simulink model "Resistive_thermal_model"  (R2017a)
settings: Solver=ode45  StartTime=0.0  StopTime=5.0  RelTol=1e-3  EnableMultiTasking=on
values from neighbouring files (symbols this model uses):
  Rth_c1 = 0.00001    (= 1e-05)    [Power_loss_calculation.m]
  Rth_c2 = 0.00001    (= 1e-05)    [Power_loss_calculation.m]
  Rth_c3 = 0.00001    (= 1e-05)    [Power_loss_calculation.m]
  Rth_heatsink = 0.01    [Power_loss_calculation.m]    (also in Thermal_plot.m = [0.005)
  Rth_jc_FWD1L = 0.12    [Power_loss_calculation.m]
  Rth_jc_FWD1U = 0.12    [Power_loss_calculation.m]
  Rth_jc_FWD2L = 0.12    [Power_loss_calculation.m]
  Rth_jc_FWD2U = 0.12    [Power_loss_calculation.m]
  Rth_jc_FWD3L = 0.12    [Power_loss_calculation.m]
  Rth_jc_FWD3U = 0.12    [Power_loss_calculation.m]
  Rth_jc_IGBT1L = 0.066    [Power_loss_calculation.m]
  Rth_jc_IGBT1U = 0.066    [Power_loss_calculation.m]
  Rth_jc_IGBT2L = 0.066    [Power_loss_calculation.m]
  Rth_jc_IGBT2U = 0.066    [Power_loss_calculation.m]
  Rth_jc_IGBT3L = 0.066    [Power_loss_calculation.m]
  Rth_jc_IGBT3U = 0.066    [Power_loss_calculation.m]
  Rth_paste = 0.015    [Power_loss_calculation.m]
libraries: fl_lib x46, nesl_utility x15
settings Model: Creator=Caner  LastModifiedBy=Caner
settings DataIOCC: LimitDataPoints=on  SaveFormat=Array
settings OptimizationCC: LifeSpan=inf
settings DebuggingCC: UnconnectedInputMsg=none  UnconnectedOutputMsg=none  UnconnectedLineMsg=none  SFUnexpectedBacktrackingDiag=warning  SFNoUnconditionalDefaultTransitionDiag=warning  SFExecutionAtInitializationDiag=none
settings HardwareCC: ProdBitPerPointer=32  ProdBitPerSizeT=32  ProdBitPerPtrDiffT=32  ProdLargestAtomicFloat=None  ProdIntDivRoundTo=Undefined  ProdEndianess=Unspecified  ProdWordSize=32  ProdHWDeviceType=32-bit Generic
settings ModelReferenceCC: PropagateSignalLabelsOutOfModel=off
settings GRTTargetCC: TargetLangStandard=C89/C90 (ANSI)  GeneratePreprocessorConditionals=Disable all
settings ConfigComp: CovMetricSettings=dw  CovHtmlReporting=on  CovSaveCumulativeToWorkspaceVar=on  CovSaveSingleToWorkspaceVar=on  CovExternalEMLEnable=off

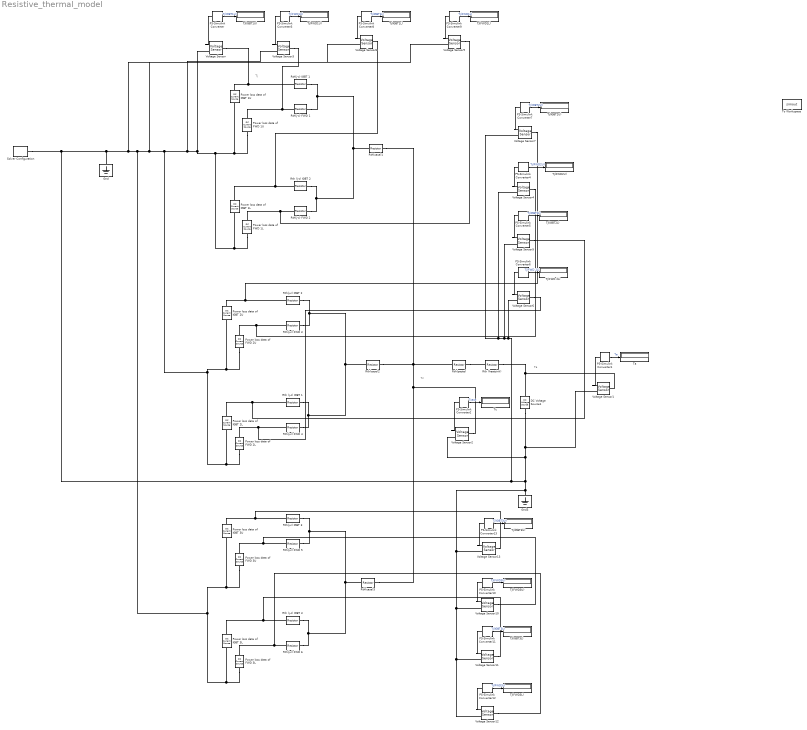
== system Resistive_thermal_model ==
  note: Ta
  note: Tc
  note: Tj
  DC Voltage Source1 : fl_lib/Electrical/Electrical Sources/DC Voltage Source  v0=40 V
  Gnd : fl_lib/Electrical/Electrical Elements/Electrical Reference
  Gnd3 : fl_lib/Electrical/Electrical Elements/Electrical Reference
  PS-Simulink Converter{,1..13} (14 alike) : nesl_utility/PS-Simulink Converter  PhysicalDomain=network_engine_domain  SubClassName=ps_output  LeftPortType=input  RightPortType=output  PseudoPeriodic=off  Frequencies=[]  Unit=1  AffineConversion=off
  Power loss data of FWD 1L : fl_lib/Electrical/Electrical Sources/DC Current Source  i0=PQ A
      settings: SourceProductName=Simscape  SourceProductBaseCode=SS
  Power loss data of FWD 1U : fl_lib/Electrical/Electrical Sources/DC Current Source  i0=PQ A
      settings: SourceProductName=Simscape  SourceProductBaseCode=SS
  Power loss data of FWD 2L : fl_lib/Electrical/Electrical Sources/DC Current Source  i0=PQ A
      settings: SourceProductName=Simscape  SourceProductBaseCode=SS
  Power loss data of FWD 2U : fl_lib/Electrical/Electrical Sources/DC Current Source  i0=PQ A
      settings: SourceProductName=Simscape  SourceProductBaseCode=SS
  Power loss data of FWD 3L : fl_lib/Electrical/Electrical Sources/DC Current Source  i0=PQ A
      settings: SourceProductName=Simscape  SourceProductBaseCode=SS
  Power loss data of FWD 3U : fl_lib/Electrical/Electrical Sources/DC Current Source  i0=PQ A
      settings: SourceProductName=Simscape  SourceProductBaseCode=SS
  Power loss data of IGBT 1L : fl_lib/Electrical/Electrical Sources/DC Current Source  i0=PD A
      settings: SourceProductName=Simscape  SourceProductBaseCode=SS
  Power loss data of IGBT 1U : fl_lib/Electrical/Electrical Sources/DC Current Source  i0=PD A
      settings: SourceProductName=Simscape  SourceProductBaseCode=SS
  Power loss data of IGBT 2L : fl_lib/Electrical/Electrical Sources/DC Current Source  i0=PD A
      settings: SourceProductName=Simscape  SourceProductBaseCode=SS
  Power loss data of IGBT 2U : fl_lib/Electrical/Electrical Sources/DC Current Source  i0=PD A
      settings: SourceProductName=Simscape  SourceProductBaseCode=SS
  Power loss data of IGBT 3L : fl_lib/Electrical/Electrical Sources/DC Current Source  i0=PD A
      settings: SourceProductName=Simscape  SourceProductBaseCode=SS
  Power loss data of IGBT 3U : fl_lib/Electrical/Electrical Sources/DC Current Source  i0=PD A
      settings: SourceProductName=Simscape  SourceProductBaseCode=SS
  Rth (heatsink) : fl_lib/Electrical/Electrical Elements/Resistor  R=Rth_heatsink Ohm  i_specify=off  i_priority=High  i=0 A  i_nominal_specify=off  i_nominal_unit=A  i_nominal_value=1  v_specify=off  v_priority=High  v=0 V  v_nominal_specify=off  v_nominal_unit=V  v_nominal_value=1
  Rth (j-c) IGBT 1 : fl_lib/Electrical/Electrical Elements/Resistor  R=Rth_jc_IGBT2L Ohm  i_specify=off  i_priority=High  i=0 A  i_nominal_specify=off  i_nominal_unit=A  i_nominal_value=1  v_specify=off  v_priority=High  v=0 V  v_nominal_specify=off  v_nominal_unit=V  v_nominal_value=1
  Rth (j-c) IGBT 2 : fl_lib/Electrical/Electrical Elements/Resistor  R=Rth_jc_IGBT1L Ohm  i_specify=off  i_priority=High  i=0 A  i_nominal_specify=off  i_nominal_unit=A  i_nominal_value=1  v_specify=off  v_priority=High  v=0 V  v_nominal_specify=off  v_nominal_unit=V  v_nominal_value=1
  Rth (j-c) IGBT 3 : fl_lib/Electrical/Electrical Elements/Resistor  R=Rth_jc_IGBT3L Ohm  i_specify=off  i_priority=High  i=0 A  i_nominal_specify=off  i_nominal_unit=A  i_nominal_value=1  v_specify=off  v_priority=High  v=0 V  v_nominal_specify=off  v_nominal_unit=V  v_nominal_value=1
  Rth(case)1 : fl_lib/Electrical/Electrical Elements/Resistor  R=Rth_c1 Ohm  i_specify=off  i_priority=High  i=0 A  i_nominal_specify=off  i_nominal_unit=A  i_nominal_value=1  v_specify=off  v_priority=High  v=0 V  v_nominal_specify=off  v_nominal_unit=V  v_nominal_value=1
  Rth(case)2 : fl_lib/Electrical/Electrical Elements/Resistor  R=Rth_c2 Ohm  i_specify=off  i_priority=High  i=0 A  i_nominal_specify=off  i_nominal_unit=A  i_nominal_value=1  v_specify=off  v_priority=High  v=0 V  v_nominal_specify=off  v_nominal_unit=V  v_nominal_value=1
  Rth(case)3 : fl_lib/Electrical/Electrical Elements/Resistor  R=Rth_c3 Ohm  i_specify=off  i_priority=High  i=0 A  i_nominal_specify=off  i_nominal_unit=A  i_nominal_value=1  v_specify=off  v_priority=High  v=0 V  v_nominal_specify=off  v_nominal_unit=V  v_nominal_value=1
  Rth(j-c) FWD 1 : fl_lib/Electrical/Electrical Elements/Resistor  R=Rth_jc_FWD1U Ohm  i_specify=off  i_priority=High  i=0 A  i_nominal_specify=off  i_nominal_unit=A  i_nominal_value=1  v_specify=off  v_priority=High  v=0 V  v_nominal_specify=off  v_nominal_unit=V  v_nominal_value=1
  Rth(j-c) FWD 2 : fl_lib/Electrical/Electrical Elements/Resistor  R=Rth_jc_FWD1L Ohm  i_specify=off  i_priority=High  i=0 A  i_nominal_specify=off  i_nominal_unit=A  i_nominal_value=1  v_specify=off  v_priority=High  v=0 V  v_nominal_specify=off  v_nominal_unit=V  v_nominal_value=1
  Rth(j-c) FWD 3 : fl_lib/Electrical/Electrical Elements/Resistor  R=Rth_jc_FWD2U Ohm  i_specify=off  i_priority=High  i=0 A  i_nominal_specify=off  i_nominal_unit=A  i_nominal_value=1  v_specify=off  v_priority=High  v=0 V  v_nominal_specify=off  v_nominal_unit=V  v_nominal_value=1
  Rth(j-c) FWD 4 : fl_lib/Electrical/Electrical Elements/Resistor  R=Rth_jc_FWD2L Ohm  i_specify=off  i_priority=High  i=0 A  i_nominal_specify=off  i_nominal_unit=A  i_nominal_value=1  v_specify=off  v_priority=High  v=0 V  v_nominal_specify=off  v_nominal_unit=V  v_nominal_value=1
  Rth(j-c) FWD 5 : fl_lib/Electrical/Electrical Elements/Resistor  R=Rth_jc_FWD3U Ohm  i_specify=off  i_priority=High  i=0 A  i_nominal_specify=off  i_nominal_unit=A  i_nominal_value=1  v_specify=off  v_priority=High  v=0 V  v_nominal_specify=off  v_nominal_unit=V  v_nominal_value=1
  Rth(j-c) FWD 6 : fl_lib/Electrical/Electrical Elements/Resistor  R=Rth_jc_FWD3L Ohm  i_specify=off  i_priority=High  i=0 A  i_nominal_specify=off  i_nominal_unit=A  i_nominal_value=1  v_specify=off  v_priority=High  v=0 V  v_nominal_specify=off  v_nominal_unit=V  v_nominal_value=1
  Rth(j-c) IGBT 1 : fl_lib/Electrical/Electrical Elements/Resistor  R=Rth_jc_IGBT1U Ohm  i_specify=off  i_priority=High  i=0 A  i_nominal_specify=off  i_nominal_unit=A  i_nominal_value=1  v_specify=off  v_priority=High  v=0 V  v_nominal_specify=off  v_nominal_unit=V  v_nominal_value=1
  Rth(j-c) IGBT 2 : fl_lib/Electrical/Electrical Elements/Resistor  R=Rth_jc_IGBT2U Ohm  i_specify=off  i_priority=High  i=0 A  i_nominal_specify=off  i_nominal_unit=A  i_nominal_value=1  v_specify=off  v_priority=High  v=0 V  v_nominal_specify=off  v_nominal_unit=V  v_nominal_value=1
  Rth(j-c) IGBT 3 : fl_lib/Electrical/Electrical Elements/Resistor  R=Rth_jc_IGBT3U Ohm  i_specify=off  i_priority=High  i=0 A  i_nominal_specify=off  i_nominal_unit=A  i_nominal_value=1  v_specify=off  v_priority=High  v=0 V  v_nominal_specify=off  v_nominal_unit=V  v_nominal_value=1
  Rth(paste) : fl_lib/Electrical/Electrical Elements/Resistor  R=Rth_paste Ohm  i_specify=off  i_priority=High  i=0 A  i_nominal_specify=off  i_nominal_unit=A  i_nominal_value=1  v_specify=off  v_priority=High  v=0 V  v_nominal_specify=off  v_nominal_unit=V  v_nominal_value=1
  Solver Configuration : nesl_utility/Solver Configuration  PhysicalDomain=network_engine_domain  SubClassName=solver  LeftPortType=input  RightPortType=generic  Accelerate=off  Tones=[]  Harmonics=[]  SimulateNoise=off  Profile=off  UseLocalSampling=off  EnableSwitchedLinearOptims=on  FrequencyDomain=off  UseCCode=off  RelTol=0.001  AbsTol=1e-06  MinStep=1e-09  ToWorkspace=off  RevertToSquareIcSolve=off  NumHomotopyIterations=100  PhasorMode=off  PhasorModeNumHarmonics=1  OverrideAbsTol=off  DoDC=off  ResidualTolerance=1e-09  UseLocalSolver=off  LocalSolverChoice=NE_BACKWARD_EULER_ADVANCER  LocalSolverSampleTime=0.001  DoFixedCost=off  MaxNonlinIter=3  MaxModeIter=2  LinearAlgebra=Sparse  DelaysMemoryBudget=1024  AutomaticFiltering=on  FilteringTimeConstant=0.001
  Ta : Display
  Tc : Display
  Tj(FWD 2L) : Display
  Tj(FWD1L) : Display
  Tj(FWD1U) : Display
  Tj(FWD2U) : Display
  Tj(FWD3L) : Display
  Tj(FWD3U) : Display
  Tj(IGBT1L) : Display
  Tj(IGBT1U) : Display
  Tj(IGBT2L) : Display
  Tj(IGBT2U) : Display
  Tj(IGBT3L) : Display
  Tj(IGBT3U) : Display
  To Workspace : ToWorkspace  VariableName=simout  SaveFormat=Timeseries  SampleTime=-1
      settings: Decimation=3
  Voltage Sensor{,1..13} (14 alike) : fl_lib/Electrical/Electrical Sensors/Voltage Sensor
  wires:
  PS-Simulink Converter/1 -> Tj(IGBT1U)/1  "Tj(IGBT1U)"
  PS-Simulink Converter1/1 -> Ta/1  "Ta"
  PS-Simulink Converter2/1 -> Tc/1  "Tcase"
  PS-Simulink Converter3/1 -> Tj(FWD1U)/1  "Tj(FWD1U)"
  PS-Simulink Converter4/1 -> Tj(FWD2U)/1  "Tj(FWD2U)"
  PS-Simulink Converter5/1 -> Tj(IGBT2L)/1  "Tj(IGBT2L)"
  PS-Simulink Converter6/1 -> Tj(FWD 2L)/1  "Tj(FWD 2L)"
  PS-Simulink Converter7/1 -> Tj(IGBT2U)/1  "Tj(IGBT2U)"
  PS-Simulink Converter8/1 -> Tj(IGBT1L)/1  "Tj(IGBT1L)"
  PS-Simulink Converter9/1 -> Tj(FWD1L)/1  "Tj(FWD1L)"
  PS-Simulink Converter11/1 -> Tj(IGBT3L)/1  "Tj(IGBT3L)"
  PS-Simulink Converter10/1 -> Tj(FWD3U)/1  "Tj(FWD3U)"
  PS-Simulink Converter13/1 -> Tj(IGBT3U)/1  "Tj(IGBT3U)"
  PS-Simulink Converter12/1 -> Tj(FWD3L)/1  "Tj(FWD3L)"
  connections:
  Power loss data of IGBT 1U/LConn1 -- Voltage Sensor/LConn1 -- Rth(j-c) IGBT 1/LConn1
  Rth (j-c) IGBT 2/RConn1 -- Rth(j-c) IGBT 1/RConn1 -- Rth(j-c) FWD 1/RConn1 -- Rth(case)1/LConn1 -- Rth(j-c) FWD 2/RConn1
  Power loss data of FWD 1U/LConn1 -- Voltage Sensor3/LConn1 -- Rth(j-c) FWD 1/LConn1
  Power loss data of FWD 1L/LConn1 -- Voltage Sensor9/LConn1 -- Rth(j-c) FWD 2/LConn1
  Power loss data of IGBT 1L/LConn1 -- Voltage Sensor8/LConn1 -- Rth (j-c) IGBT 2/LConn1
  Rth(j-c) IGBT 2/RConn1 -- Rth (j-c) IGBT 1/RConn1 -- Rth(j-c) FWD 4/RConn1 -- Rth(case)2/LConn1 -- Rth(j-c) FWD 3/RConn1
  Power loss data of FWD 2U/LConn1 -- Voltage Sensor4/LConn1 -- Rth(j-c) FWD 3/LConn1
  Power loss data of IGBT 2U/LConn1 -- Voltage Sensor7/LConn1 -- Rth(j-c) IGBT 2/LConn1
  Rth(case)2/RConn1 -- Rth(case)3/RConn1 -- Voltage Sensor2/LConn1 -- Rth(case)1/RConn1 -- Rth(paste)/LConn1
  Power loss data of IGBT 2L/LConn1 -- Voltage Sensor5/LConn1 -- Rth (j-c) IGBT 1/LConn1
  Power loss data of FWD 2L/LConn1 -- Voltage Sensor6/LConn1 -- Rth(j-c) FWD 4/LConn1
  Rth(j-c) IGBT 3/RConn1 -- Rth (j-c) IGBT 3/RConn1 -- Rth(j-c) FWD 6/RConn1 -- Rth(case)3/LConn1 -- Rth(j-c) FWD 5/RConn1
  Power loss data of FWD 3U/LConn1 -- Voltage Sensor10/LConn1 -- Rth(j-c) FWD 5/LConn1
  Power loss data of IGBT 3U/LConn1 -- Voltage Sensor13/LConn1 -- Rth(j-c) IGBT 3/LConn1
  Power loss data of IGBT 3L/LConn1 -- Voltage Sensor11/LConn1 -- Rth (j-c) IGBT 3/LConn1
  Power loss data of FWD 3L/LConn1 -- Voltage Sensor12/LConn1 -- Rth(j-c) FWD 6/LConn1
  Rth(paste)/RConn1 -- Rth (heatsink)/LConn1
  Rth (heatsink)/RConn1 -- Voltage Sensor1/LConn1 -- DC Voltage Source1/LConn1
  Voltage Sensor/RConn1 -- PS-Simulink Converter/LConn1
  Voltage Sensor1/RConn1 -- PS-Simulink Converter1/LConn1
  Voltage Sensor2/RConn1 -- PS-Simulink Converter2/LConn1
  Voltage Sensor3/RConn1 -- PS-Simulink Converter3/LConn1
  Voltage Sensor4/RConn1 -- PS-Simulink Converter4/LConn1
  Voltage Sensor5/RConn1 -- PS-Simulink Converter5/LConn1
  Voltage Sensor6/RConn1 -- PS-Simulink Converter6/LConn1
  Voltage Sensor7/RConn1 -- PS-Simulink Converter7/LConn1
  Voltage Sensor8/RConn1 -- PS-Simulink Converter8/LConn1
  Voltage Sensor9/RConn1 -- PS-Simulink Converter9/LConn1
  Voltage Sensor13/RConn1 -- PS-Simulink Converter13/LConn1
  Voltage Sensor12/RConn1 -- PS-Simulink Converter12/LConn1
  Voltage Sensor10/RConn1 -- PS-Simulink Converter10/LConn1
  Voltage Sensor11/RConn1 -- PS-Simulink Converter11/LConn1
  Voltage Sensor13/RConn2 -- Voltage Sensor10/RConn2 -- Voltage Sensor11/RConn2 -- Voltage Sensor12/RConn2 -- Gnd3/LConn1 -- Voltage Sensor6/RConn2 -- Voltage Sensor5/RConn2 -- Voltage Sensor4/RConn2 -- Voltage Sensor7/RConn2 -- Voltage Sensor8/RConn2 -- Power loss data of IGBT 3L/RConn1 -- Power loss data of FWD 3L/RConn1 -- Power loss data of FWD 3U/RConn1 -- Power loss data of IGBT 3U/RConn1 -- Voltage Sensor9/RConn2 -- Voltage Sensor3/RConn2 -- Voltage Sensor/RConn2 -- Power loss data of IGBT 1L/RConn1 -- Power loss data of FWD 1L/RConn1 -- Power loss data of FWD 1U/RConn1 -- Power loss data of IGBT 1U/RConn1 -- Power loss data of IGBT 2L/RConn1 -- Power loss data of FWD 2L/RConn1 -- Power loss data of FWD 2U/RConn1 -- Power loss data of IGBT 2U/RConn1 -- Gnd/LConn1 -- Solver Configuration/RConn1 -- DC Voltage Source1/RConn1 -- Voltage Sensor1/RConn2 -- Voltage Sensor2/RConn2
